simulink model "ProdSys_Push"  (R2015b)
settings: Solver=ode45  StartTime=0.0  StopTime=100000  RelTol=1e-3
PostLoadFcn:
  | set_param(gcs, 'Location', [0 0 1750 500])
libraries: simeventslib x3, simulink x1
settings Model: Creator=tsprock3  LastModifiedBy=tsprock3
settings DataIOCC: SaveFormat=Array
settings OptimizationCC: ExpressionDepthLimit=2147483647  SimCompilerOptimization=on
settings DebuggingCC: UnderspecifiedInitializationDetection=Classic  MergeDetectMultiDrivingBlocksExec=none  SolverPrmCheckMsg=warning  FcnCallInpInsideContextMsg=EnableAllAsWarning  StateNameClashWarn=warning
settings HardwareCC: ProdBitPerPointer=32  ProdLargestAtomicFloat=None  ProdIntDivRoundTo=Undefined  ProdEndianess=Unspecified  ProdWordSize=32  ProdHWDeviceType=32-bit Generic
settings GRTTargetCC: GeneratePreprocessorConditionals=Disable all
settings ConfigComp: CovModelRefEnable=Off

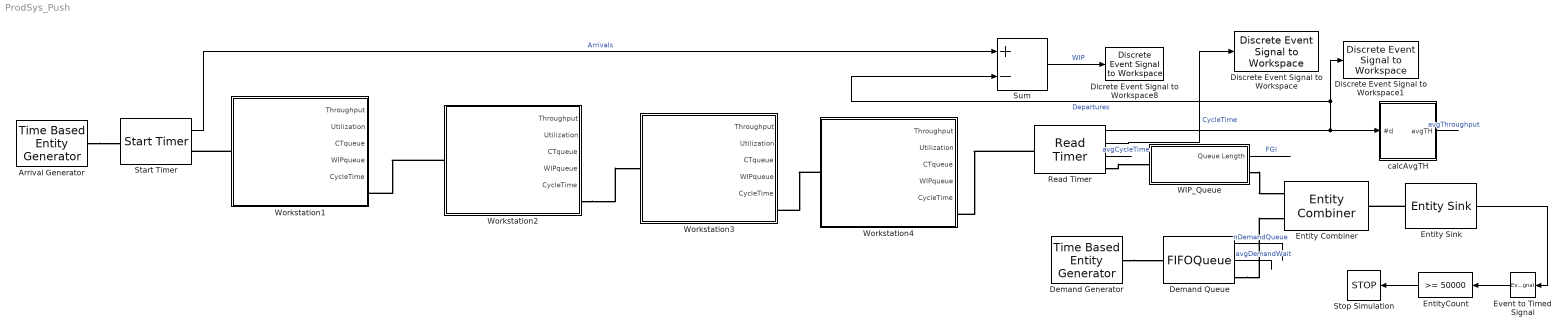
== system ProdSys_Push ==
  Arrival Generator : TimeBasedEntityGenerator  Distribution=Exponential  Period=1/0.37  Mean=1/0.4
  Demand Generator : TimeBasedEntityGenerator  Distribution=Exponential  Period=1/0.37  Mean=1/0.4
  Demand Queue : FIFOQueue  Capacity=100  StatNumberInBlock=on  StatAverageWait=on
      settings: OutputPortMap=o1,o2
  Dicrete Event Signal to Workspace8 : simeventslib/SimEvents Sinks/Discrete Event Signal to Workspace  VariableName=WIP  SaveFormat=Structure With Time  isMonitorOnly=off  isRecordIC=off
  Discrete Event Signal to Workspace : simeventslib/SimEvents Sinks/Discrete Event Signal to Workspace  VariableName=CycleTime  SaveFormat=Structure With Time  isMonitorOnly=off  isRecordIC=off
  Discrete Event Signal to Workspace1 : simeventslib/SimEvents Sinks/Discrete Event Signal to Workspace  VariableName=Departures  SaveFormat=Structure With Time  isMonitorOnly=off  isRecordIC=off
  Entity Combiner : EntityCombiner  NumberInputPorts=2  RetainComponentEntities=off
  Entity Sink : EntitySink  StatNumberArrived=on
  EntityCount : simulink/Logic and Bit Operations/Compare To Constant  relop=>=  const=50000  OutDataTypeStr=boolean
  Event to Timed Signal : EventToTimedSignal
  Read Timer : ReadTimer  TimerTag=CycleTime  StatNumberDeparted=on  StatTimeElapsed=on  StatAverageTimeElapsed=on
      settings: OutputPortMap=o0,o2,o3
  Start Timer : StartTimer  TimerTag=CycleTime  TimerStartedOption=Restart  StatNumberDeparted=on
  Stop Simulation : Stop
  Sum : Sum  Inputs=|+-
  WIP_Queue : Subsystem  mask{NumberOfEventsPerPeriod=10}
      mask prompts: NumberOfEventsPerPeriod "W0"
      mask TypeOptions NumberOfEventsPerPeriod: Generate/NumberOfEventsPerPeriod
  Workstation1 : Subsystem  mask{NumberOfServers=1, Capacity=inf}
      mask prompts: NumberOfServers "m = Number of Parallel Servers"; Capacity "b = buffer size"
      mask TypeOptions NumberOfServers: N-Server/NumberOfServers
      mask TypeOptions Capacity: FIFO Queue/Capacity
  Workstation2 : Subsystem  mask{NumberOfServers=1, Capacity=inf}
      mask prompts: NumberOfServers "m = Number of Parallel Servers"; Capacity "b = buffer size"
      mask TypeOptions NumberOfServers: N-Server/NumberOfServers
      mask TypeOptions Capacity: FIFO Queue/Capacity
  Workstation3 : Subsystem  mask{NumberOfServers=1, Capacity=inf}
      mask prompts: NumberOfServers "m = Number of Parallel Servers"; Capacity "b = buffer size"
      mask TypeOptions NumberOfServers: N-Server/NumberOfServers
      mask TypeOptions Capacity: FIFO Queue/Capacity
  Workstation4 : Subsystem  mask{NumberOfServers=1, Capacity=inf}
      mask prompts: NumberOfServers "m = Number of Parallel Servers"; Capacity "b = buffer size"
      mask TypeOptions NumberOfServers: N-Server/NumberOfServers
      mask TypeOptions Capacity: FIFO Queue/Capacity
  calcAvgTH : Subsystem
  wires:
  Read Timer/2 -> Discrete Event Signal to Workspace/1  "CycleTime"
  Sum/1 -> Dicrete Event Signal to Workspace8/1  "WIP"
  Start Timer/1 -> Sum/1  "Arrivals"
  Read Timer/1 -> Discrete Event Signal to Workspace1/1, Sum/2, calcAvgTH/1(#d)  "Departures"
  Demand Queue/1 -> ?  "nDemandQueue"
  Demand Queue/2 -> ?  "avgDemandWait"
  WIP_Queue/1(Queue Length) -> ?  "FGI"
  calcAvgTH/1(avgTH) -> ?  "avgThroughput"
  Read Timer/3 -> ?  "avgCycleTime"
  Entity Sink/1 -> Event to Timed Signal/1
  EntityCount/1 -> Stop Simulation/1
  Event to Timed Signal/1 -> EntityCount/1
  connections:
  Workstation1/LConn1 -- Start Timer/RConn1
  Arrival Generator/RConn1 -- Start Timer/LConn1
  Read Timer/LConn1 -- Workstation4/RConn1
  Demand Queue/RConn1 -- Entity Combiner/LConn2
  Demand Generator/RConn1 -- Demand Queue/LConn1
  WIP_Queue/RConn1 -- Entity Combiner/LConn1
  Entity Sink/LConn1 -- Entity Combiner/RConn1
  Read Timer/RConn1 -- WIP_Queue/LConn1
  Workstation2/LConn1 -- Workstation1/RConn1
  Workstation4/LConn1 -- Workstation3/RConn1
  Workstation2/RConn1 -- Workstation3/LConn1

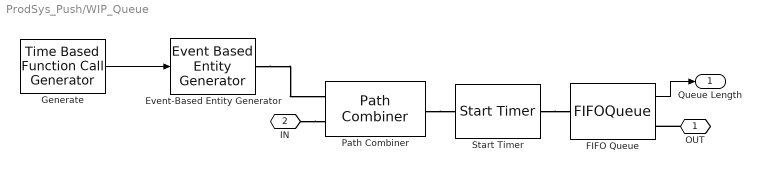
== system ProdSys_Push/WIP_Queue ==
  Event-Based Entity Generator : EventBasedEntityGenerator  GenerateEntitiesUpon=Function call from port fcn
  FIFO Queue : FIFOQueue  StatNumberInBlock=on
      settings: OutputPortMap=o1
  Generate : TimeBasedFunctionCallGenerator  EventGenerationMode=Only at simulation start  NumberOfEventsPerPeriod=NumberOfEventsPerPeriod
  Path Combiner : PathCombiner  NumberInputPorts=2
  Start Timer : StartTimer  TimerStartedOption=Restart
  OUT : PMIOPort  Port=1  Side=Right
  IN : PMIOPort  Port=2  Side=Left
  Queue Length : Outport
  wires:
  Generate/1 -> Event-Based Entity Generator/1
  FIFO Queue/1 -> Queue Length/1
  connections:
  Start Timer/RConn1 -- FIFO Queue/LConn1
  Path Combiner/RConn1 -- Start Timer/LConn1
  OUT/RConn1 -- FIFO Queue/RConn1
  IN/RConn1 -- Path Combiner/LConn2
  Event-Based Entity Generator/RConn1 -- Path Combiner/LConn1

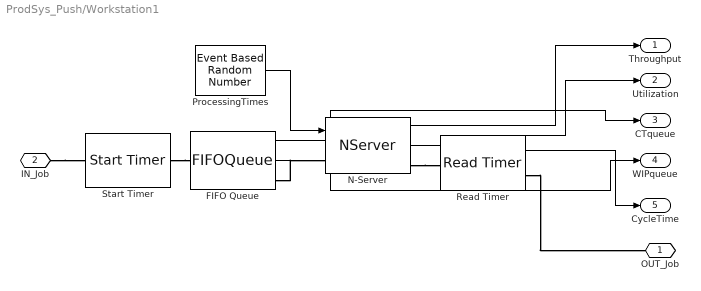
== system ProdSys_Push/Workstation1 ==
  FIFO Queue : FIFOQueue  Capacity=Capacity  StatAverageWait=on  StatAverageQueueLength=on
      settings: OutputPortMap=o2,o3
  N-Server : NServer  NumberOfServers=NumberOfServers  ServiceTimeFrom=Signal port t  StatNumberDeparted=on  StatUtilization=on
      settings: OutputPortMap=o0,o5
  ProcessingTimes : EventBasedRandomNumber  meanExp=2  meanNorm=5  stdNorm=2  Seed=1
  Read Timer : ReadTimer  TimerTag=WorkstationCycleTime  StatAverageTimeElapsed=on
      settings: OutputPortMap=o3
  Start Timer : StartTimer  TimerTag=WorkstationCycleTime  TimerStartedOption=Restart
  OUT_Job : PMIOPort  Port=1  Side=Right
  IN_Job : PMIOPort  Port=2  Side=Left
  Throughput : Outport
  Utilization : Outport  Port=2
  CTqueue : Outport  Port=3
  WIPqueue : Outport  Port=4
  CycleTime : Outport  Port=5
  wires:
  ProcessingTimes/1 -> N-Server/1
  N-Server/1 -> Throughput/1
  N-Server/2 -> Utilization/1
  FIFO Queue/1 -> CTqueue/1
  FIFO Queue/2 -> WIPqueue/1
  Read Timer/1 -> CycleTime/1
  connections:
  FIFO Queue/RConn1 -- N-Server/LConn1
  IN_Job/RConn1 -- Start Timer/LConn1
  Start Timer/RConn1 -- FIFO Queue/LConn1
  N-Server/RConn1 -- Read Timer/LConn1
  Read Timer/RConn1 -- OUT_Job/RConn1

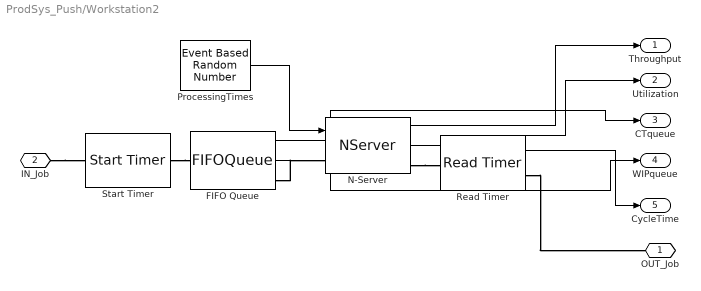
== system ProdSys_Push/Workstation2 ==
  FIFO Queue : FIFOQueue  Capacity=Capacity  StatAverageWait=on  StatAverageQueueLength=on
      settings: OutputPortMap=o2,o3
  N-Server : NServer  NumberOfServers=NumberOfServers  ServiceTimeFrom=Signal port t  StatNumberDeparted=on  StatUtilization=on
      settings: OutputPortMap=o0,o5
  ProcessingTimes : EventBasedRandomNumber  meanExp=2  meanNorm=5  stdNorm=2  Seed=2
  Read Timer : ReadTimer  TimerTag=WorkstationCycleTime  StatAverageTimeElapsed=on
      settings: OutputPortMap=o3
  Start Timer : StartTimer  TimerTag=WorkstationCycleTime  TimerStartedOption=Restart
  OUT_Job : PMIOPort  Port=1  Side=Right
  IN_Job : PMIOPort  Port=2  Side=Left
  Throughput : Outport
  Utilization : Outport  Port=2
  CTqueue : Outport  Port=3
  WIPqueue : Outport  Port=4
  CycleTime : Outport  Port=5
  wires:
  ProcessingTimes/1 -> N-Server/1
  N-Server/1 -> Throughput/1
  N-Server/2 -> Utilization/1
  FIFO Queue/1 -> CTqueue/1
  FIFO Queue/2 -> WIPqueue/1
  Read Timer/1 -> CycleTime/1
  connections:
  FIFO Queue/RConn1 -- N-Server/LConn1
  IN_Job/RConn1 -- Start Timer/LConn1
  Start Timer/RConn1 -- FIFO Queue/LConn1
  N-Server/RConn1 -- Read Timer/LConn1
  Read Timer/RConn1 -- OUT_Job/RConn1

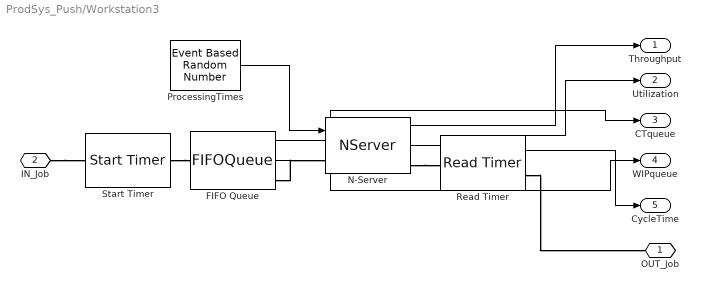
== system ProdSys_Push/Workstation3 ==
  FIFO Queue : FIFOQueue  Capacity=Capacity  StatAverageWait=on  StatAverageQueueLength=on
      settings: OutputPortMap=o2,o3
  N-Server : NServer  NumberOfServers=NumberOfServers  ServiceTimeFrom=Signal port t  StatNumberDeparted=on  StatUtilization=on
      settings: OutputPortMap=o0,o5
  ProcessingTimes : EventBasedRandomNumber  meanExp=2  meanNorm=5  stdNorm=2  Seed=3
  Read Timer : ReadTimer  TimerTag=WorkstationCycleTime  StatAverageTimeElapsed=on
      settings: OutputPortMap=o3
  Start Timer : StartTimer  TimerTag=WorkstationCycleTime  TimerStartedOption=Restart
  OUT_Job : PMIOPort  Port=1  Side=Right
  IN_Job : PMIOPort  Port=2  Side=Left
  Throughput : Outport
  Utilization : Outport  Port=2
  CTqueue : Outport  Port=3
  WIPqueue : Outport  Port=4
  CycleTime : Outport  Port=5
  wires:
  ProcessingTimes/1 -> N-Server/1
  N-Server/1 -> Throughput/1
  N-Server/2 -> Utilization/1
  FIFO Queue/1 -> CTqueue/1
  FIFO Queue/2 -> WIPqueue/1
  Read Timer/1 -> CycleTime/1
  connections:
  FIFO Queue/RConn1 -- N-Server/LConn1
  IN_Job/RConn1 -- Start Timer/LConn1
  Start Timer/RConn1 -- FIFO Queue/LConn1
  N-Server/RConn1 -- Read Timer/LConn1
  Read Timer/RConn1 -- OUT_Job/RConn1

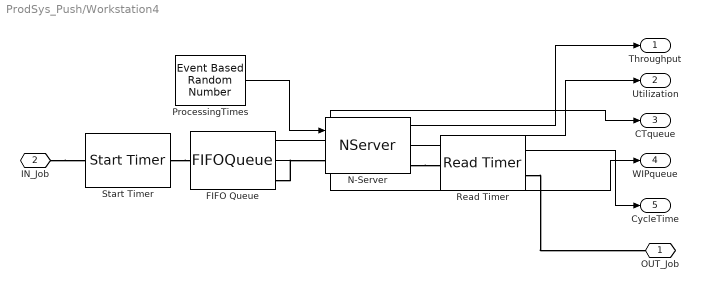
== system ProdSys_Push/Workstation4 ==
  FIFO Queue : FIFOQueue  Capacity=Capacity  StatAverageWait=on  StatAverageQueueLength=on
      settings: OutputPortMap=o2,o3
  N-Server : NServer  NumberOfServers=NumberOfServers  ServiceTimeFrom=Signal port t  StatNumberDeparted=on  StatUtilization=on
      settings: OutputPortMap=o0,o5
  ProcessingTimes : EventBasedRandomNumber  meanExp=2  meanNorm=5  stdNorm=2  Seed=4
  Read Timer : ReadTimer  TimerTag=WorkstationCycleTime  StatAverageTimeElapsed=on
      settings: OutputPortMap=o3
  Start Timer : StartTimer  TimerTag=WorkstationCycleTime  TimerStartedOption=Restart
  OUT_Job : PMIOPort  Port=1  Side=Right
  IN_Job : PMIOPort  Port=2  Side=Left
  Throughput : Outport
  Utilization : Outport  Port=2
  CTqueue : Outport  Port=3
  WIPqueue : Outport  Port=4
  CycleTime : Outport  Port=5
  wires:
  ProcessingTimes/1 -> N-Server/1
  N-Server/1 -> Throughput/1
  N-Server/2 -> Utilization/1
  FIFO Queue/1 -> CTqueue/1
  FIFO Queue/2 -> WIPqueue/1
  Read Timer/1 -> CycleTime/1
  connections:
  FIFO Queue/RConn1 -- N-Server/LConn1
  IN_Job/RConn1 -- Start Timer/LConn1
  Start Timer/RConn1 -- FIFO Queue/LConn1
  N-Server/RConn1 -- Read Timer/LConn1
  Read Timer/RConn1 -- OUT_Job/RConn1

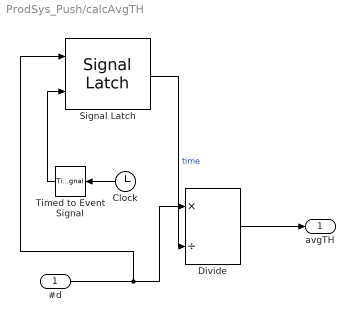
== system ProdSys_Push/calcAvgTH ==
  #d : Inport
  Clock : Clock
  Divide : Product  Inputs=*/
  Signal Latch : SignalLatch  ReadMemoryUpon=Write to memory event
      settings: InputPortMap=u0,u2  OutputPortMap=o2
  Timed to Event Signal : TimedToEventSignal
  avgTH : Outport
  wires:
  #d/1 -> Signal Latch/1, Divide/1
  Timed to Event Signal/1 -> Signal Latch/2
  Signal Latch/1 -> Divide/2  "time"
  Clock/1 -> Timed to Event Signal/1
  Divide/1 -> avgTH/1
